simulink model "IBDC_DAB_SC"  (R2020b)
settings: Solver=VariableStepAuto  StartTime=0.0  StopTime=0.2  MaxStep=5.0E-7  RelTol=1e-3
values from neighbouring files (symbols this model uses):
  L = 19.5e-6    (= 1.95e-05)    [Initialize.m]
  P = 1/f    (= 4e-06)    [Initialize.m]
  R_load = 115.8    [Initialize.m]
  Sample = 1e-8    (= 1e-08)    [Initialize.m]
  Vref = 340    [Initialize.m]
libraries: powerlib x32, powerlib_meascontrol x6, pid_lib x2, electricdrivelib x1
settings Model: Creator=reigs  LastModifiedBy=reigs
settings SolverCC: DecoupledContinuousIntegration=on

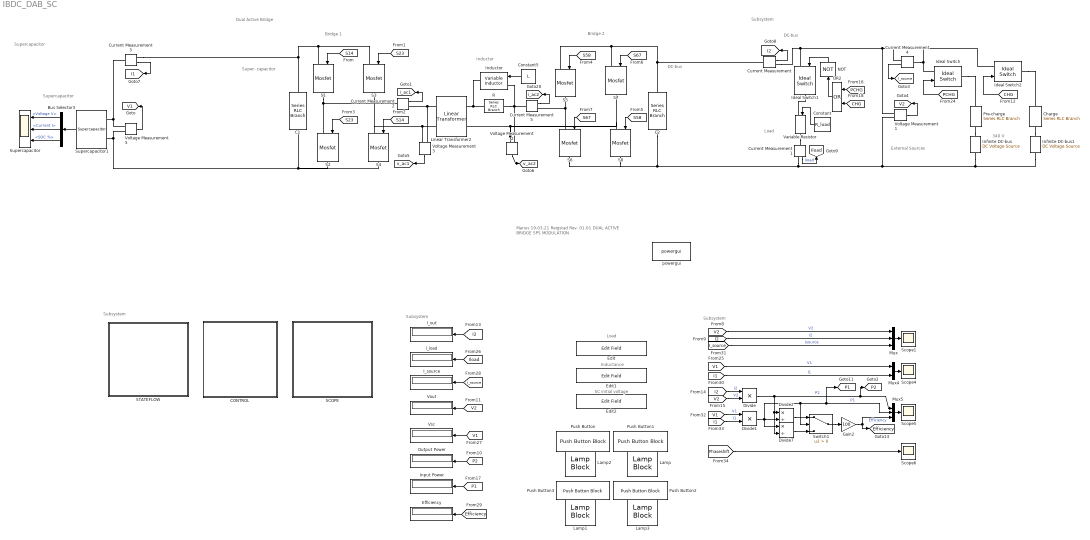
== system IBDC_DAB_SC ==
  note: Subsystem
  note: Dual Active Bridge
  note: Subsystem
  note: Subsystem
  note: Subsystem
  note: Supercapacitor
  note: Marius 19.03.21
      | Reigstad Rev. 01.01
      |
      | DUAL ACTIVE BRIDGE
      | SPS MODULATION
  note: Supercapacitor
  note: SC initial voltage
  note: Inductance
  note: Load
  note: Inductor
  note: Bridge 1
  note: Bridge 2
  note: DC-bus
  note: Super-
      | capacitor
  note: 340 V
  note: DC-bus
  note: External Sources
  note: Load
  " Inductor" : powerlib/Elements/Variable Inductor  methode=Backward Euler  Labsmin=1e-6  Initialize=off  iL0=0  L0=1e-3  Vl0=0
      settings: SourceProductBaseCode=PS
  Bus Selector3 : BusSelector  OutputSignals=Voltage V,Current I,SOC %
  C1 : powerlib/Elements/Series RLC Branch  LConnTagsString=__new0  RConnTagsString=__new0  BranchType=RC  Resistance=0.0032  Inductance=1e-3  SetiL0=off  InitialCurrent=0  Capacitance=500e-6  Setx0=on  InitialVoltage=Vsc  Measurements=None
  C2 : powerlib/Elements/Series RLC Branch  LConnTagsString=__new0  RConnTagsString=__new0  BranchType=RC  Resistance=0.0000001  Inductance=1e-3  SetiL0=off  InitialCurrent=0  Capacitance=54e-6  Setx0=off  InitialVoltage=340  Measurements=None
  CONTROL : Subsystem
  Charge : powerlib/Elements/Series RLC Branch  LConnTagsString=__new0  RConnTagsString=__new0  BranchType=R  Resistance=2  Inductance=1e-3  SetiL0=off  InitialCurrent=0  Capacitance=500e-6  Setx0=off  InitialVoltage=340  Measurements=None
  Constant : Constant  Value=R_load
  Constant5 : Constant  Value=L
  Current Measurement{,1..5} (6 alike) : powerlib/Measurements/Current Measurement  PhasorSimulation=off  OutputType=Complex  PSBequivalent=0
  Divide : Product  Inputs=**
  Divide1 : Product  Inputs=**
  Divide2 : Product  Inputs=*/
  Divide7 : Product  Inputs=*/
  Edit : EditField  LabelPosition=Hide  ShowInitialText=on  Alignment=Center
  Edit1 : EditField  LabelPosition=Hide  ShowInitialText=on  Alignment=Center
  Edit2 : EditField  LabelPosition=Hide  ShowInitialText=on  Alignment=Center
  Efficiency : Display
  Gain2 : Gain  Gain=100
  I_load : Display
  I_out : Display
  I_source : Display
  Ideal Switch : powerlib/Power Electronics/Ideal Switch  Ron=0.001  Lon=0  IC=0  Rs=1e5  Cs=inf  Measurements=off
  Ideal Switch1 : powerlib/Power Electronics/Ideal Switch  Ron=0.001  Lon=0  IC=0  Rs=1e5  Cs=inf  Measurements=off
  Ideal Switch2 : powerlib/Power Electronics/Ideal Switch  Ron=0.001  Lon=0  IC=0  Rs=1e5  Cs=inf  Measurements=off
  Infinite DC-bus : powerlib/Electrical Sources/DC Voltage Source  Amplitude=Vref  Measurements=None
  Infinite DC-bus1 : powerlib/Electrical Sources/DC Voltage Source  Amplitude=Vref  Measurements=None
  Input Power : Display
  Lamp{,1..3} (4 alike) : LampBlock
  Linear Transformer2 : powerlib/Elements/Linear Transformer  UNITS=SI  NominalPower=[2000 250000]  winding1=[180 0.0324 8.2505e-07]  winding2=[340 0.1156 2.9438e-06]  ThreeWindings=off  winding3=[3.15e+05 99225 2.5267]  RmLm=[8100 0.0051565]  Measurements=None  DataType=on
  Mux : Mux  Inputs=3
  Mux4 : Mux  Inputs=2
  Mux5 : Mux  Inputs=3
  NOT : Logic  Operator=NOT  IconShape=distinctive  AllPortsSameDT=off  OutDataTypeStr=boolean
  OR2 : Logic  Operator=OR  IconShape=distinctive  AllPortsSameDT=off  OutDataTypeStr=boolean
  Output Power : Display
  Pre-charge : powerlib/Elements/Series RLC Branch  LConnTagsString=__new0  RConnTagsString=__new0  BranchType=R  Resistance=30  Inductance=1e-3  SetiL0=off  InitialCurrent=0  Capacitance=500e-6  Setx0=off  InitialVoltage=340  Measurements=None
  Push Button : PushButtonBlock  ButtonText=STOP
  Push Button1 : PushButtonBlock  ButtonText=CHARGE
  Push Button2 : PushButtonBlock  ButtonText=STABILIZE
  Push Button3 : PushButtonBlock  ButtonText=PRECHARGE
  R : powerlib/Elements/Series RLC Branch  LConnTagsString=__new0  RConnTagsString=__new0  BranchType=R  Resistance=1e9  Inductance=1e-3  SetiL0=off  InitialCurrent=0  Capacitance=54.3e-6  Setx0=on  InitialVoltage=167  Measurements=None
  S{1..8} (8 alike) : powerlib/Power Electronics/Mosfet  Ron=ron_mosfet_pri  Lon=0  Rd=ron_body_diode_pri  Vfd=vf_body_diode_pri  IC=0  Rs=1e5  Cs=inf  Measurements=off
  SCOPE : Subsystem
  STATEFLOW : Subsystem
  Scope{1,4..6} (4 alike) : Scope
  Supercapacitor : Scope  NumInputPorts=3
  Supercapacitor1 : electricdrivelib/Extra Sources/Supercapacitor  C=5  Rdc=230.4e-3  Voltage=180  Ns=72  Np=1  Vinit=Vsc  Temp=25  PresetModel=off  EstParam=off  Nc=1  r=1e-9  epsilon=6.0208e-10  Ich=10  Vstern="[0.161  2.7  7.8]"  Self_dis=on  Ioc=10  Vself="[48  47.8  47.06  44.65]"  demandeplot=off  I="[5.55  6.25  ]"  Units=sec  Vmax=0  If=0  deltaV=0  alpha=0  sec=0
      settings: SourceProductBaseCode=PS
  Switch1 : Switch  Criteria=u2 > Threshold
  Variable Resistor : powerlib/Elements/Variable Resistor  Rabsmin=1e-3
      settings: SourceProductBaseCode=PS
  Voltage Measurement{1..3,5} (4 alike) : powerlib/Measurements/Voltage Measurement  PhasorSimulation=off  OutputType=Complex  PSBequivalent=0
  Vout : Display
  Vsc : Display
  powergui : powerlib/powergui  Priority=1  SimulationMode=Discrete  SampleTime=1e-8  frequency=60  Iterations=50  frequencyindice=0  Pbase=100e6  ErrMax=1e-4  UnitsV=kV  UnitsW=MW  buscounter=0  FunctionMessages=off  echomessages=off  EnableUseOfTLC=off  CurrentSourceSwitches=off  DisableSnubberDevices=off  DisableRonSwitches=off  DisableVfSwitches=off  DisplayEquations=off  AutomaticDiscreteSolvers=off  SolverType=Tustin/Backward Euler (TBE)  Interpol=off  ExternalGateDelay=off  methode=off  Ts=100  x0status=blocks  SPID=on  SwTol=0  HookPort=off  NonlinearTolerance=1e-4  nMaxIteration=100  ContinueOnMaxIteration=off  RestoreLinks=warning  ResistiveCurrentMeasurement=off  Frange=[0:2:500]  Ylog=off  Xlog=on  ShowGrid=off  save=off  variable=ZData  structure=0  ZoomFFT=off  StartTime=0.0  cycles=1  DisplayStyle=1  fundamental=60  FreqAxis=off  MaxFrequency=1000  frequencyindicesteady=1  RmsSteady=1  display=off
  tag scope: Efficiency=global, I1=global, I2=global, I_source=global, Iload=global, P1=global, P2=global, V1=global, V2=global, i_ac1=global, i_ac2=global, v_ac1=global, v_ac2=global
  wires:
  Current Measurement3/1 -> [I1]
  Supercapacitor1/1 -> Bus Selector3/1
  Voltage Measurement5/1 -> [V1]
  Bus Selector3/3 -> Supercapacitor/3  "<SOC %>"
  Bus Selector3/1 -> Supercapacitor/1  "<Voltage V>"
  Bus Selector3/2 -> Supercapacitor/2  "<Current I>"
  [P2] -> Output Power/1
  [Efficiency] -> Efficiency/1
  [I_source] -> I_source/1
  [V2] -> Vout/1
  [P1] -> Input Power/1
  [I2] -> I_out/1
  [Iload] -> I_load/1
  [V1] -> Vsc/1
  [I2] -> Divide/1  "I2"
  [I1] -> Divide1/2  "I1"
  Mux4/1 -> Scope4/1
  [I_source] -> Mux/3  "Isource"
  [I2] -> Mux/2  "I2"
  [Phaseshift] -> Scope6/1
  [V2] -> Mux/1  "V2"
  [I1] -> Mux4/2  "I1"
  Divide1/1 -> Switch1/2, Mux5/2, [P1], Divide2/2, Divide7/1  "P1"
  Mux/1 -> Scope1/1
  [V2] -> Divide/2  "V2"
  [V1] -> Mux4/1  "V1"
  Gain2/1 -> Mux5/3, [Efficiency]  "Efficiency"
  [V1] -> Divide1/1  "V1"
  Mux5/1 -> Scope5/1
  Divide/1 -> Divide7/2, Divide2/1, Mux5/1, [P2]  "P2"
  Switch1/1 -> Gain2/1
  Divide7/1 -> Switch1/3
  Divide2/1 -> Switch1/1
  [S58] -> S5/1
  [S14] -> S4/1
  [S67] -> S6/1
  Voltage Measurement2/1 -> [v_ac2]
  Voltage Measurement3/1 -> [v_ac1]
  [S23] -> S3/1
  [S67] -> S7/1
  [S58] -> S8/1
  Current Measurement2/1 -> [i_ac1]
  Current Measurement5/1 -> [i_ac2]
  [S23] -> S2/1
  [S14] -> S1/1
  Constant5/1 -> " Inductor"/1
  NOT/1 -> Ideal Switch1/1
  Current Measurement4/1 -> [I_source]
  [PCHG] -> OR2/1
  OR2/1 -> NOT/1
  [PCHG] -> Ideal Switch/1
  [CHG] -> OR2/2
  [CHG] -> Ideal Switch2/1
  Constant/1 -> Variable Resistor/1
  Voltage Measurement1/1 -> [V2]
  Current Measurement/1 -> [I2]
  Current Measurement1/1 -> [Iload]  "Iload"
  connections:
  Current Measurement3/LConn1 -- Voltage Measurement5/LConn1 -- Supercapacitor1/LConn1
  S1/RConn1 -- S2/LConn1 -- Current Measurement2/LConn1
  S1/LConn1 -- Current Measurement3/RConn1 -- C1/LConn1 -- S3/LConn1
  Voltage Measurement3/LConn2 -- Linear Transformer2/LConn2 -- S3/RConn1 -- S4/LConn1
  Supercapacitor1/LConn2 -- S4/RConn1 -- S2/RConn1 -- C1/RConn1 -- Voltage Measurement5/LConn2
  Current Measurement5/LConn1 -- R/LConn1 -- Voltage Measurement2/LConn1 -- " Inductor"/LConn1
  R/RConn1 -- " Inductor"/RConn1 -- Linear Transformer2/RConn1
  S6/LConn1 -- S5/RConn1 -- Current Measurement5/RConn1
  Voltage Measurement2/LConn2 -- S8/LConn1 -- S7/RConn1 -- Linear Transformer2/RConn2
  Voltage Measurement3/LConn1 -- Linear Transformer2/LConn1 -- Current Measurement2/RConn1
  Infinite DC-bus/LConn1 -- Infinite DC-bus1/LConn1 -- S6/RConn1 -- S8/RConn1 -- C2/RConn1 -- Current Measurement1/RConn1 -- Voltage Measurement1/LConn2
  Charge/RConn1 -- Infinite DC-bus1/RConn1
  C2/LConn1 -- Current Measurement/LConn1 -- S7/LConn1 -- S5/LConn1
  Ideal Switch1/RConn1 -- Variable Resistor/LConn1
  Current Measurement4/LConn1 -- Ideal Switch/LConn1 -- Ideal Switch2/LConn1
  Variable Resistor/RConn1 -- Current Measurement1/LConn1
  Pre-charge/RConn1 -- Infinite DC-bus/RConn1
  Ideal Switch/RConn1 -- Pre-charge/LConn1
  Ideal Switch2/RConn1 -- Charge/LConn1
  Current Measurement/RConn1 -- Ideal Switch1/LConn1 -- Voltage Measurement1/LConn1 -- Current Measurement4/RConn1

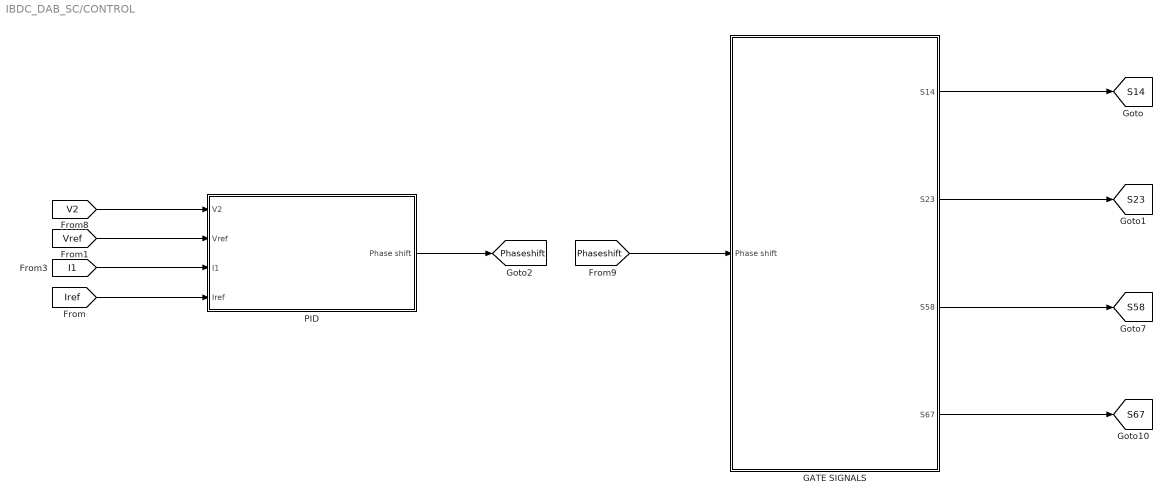
== system IBDC_DAB_SC/CONTROL ==
  GATE SIGNALS : Subsystem
  PID : Subsystem
  tag scope: Phaseshift=global, S14=global, S23=global, S58=global, S67=global
  wires:
  [Phaseshift] -> GATE SIGNALS/1(Phase shift)
  [V2] -> PID/1(V2)
  [Vref] -> PID/2(Vref)
  GATE SIGNALS/1(S14) -> [S14]
  GATE SIGNALS/2(S23) -> [S23]
  GATE SIGNALS/3(S58) -> [S58]
  GATE SIGNALS/4(S67) -> [S67]
  PID/1(Phase shift) -> [Phaseshift]
  [I1] -> PID/3(I1)
  [Iref] -> PID/4(Iref)

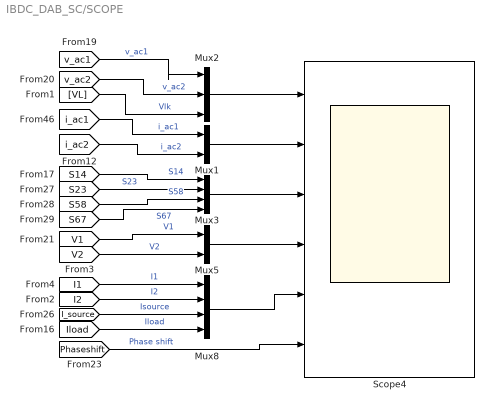
== system IBDC_DAB_SC/SCOPE ==
  Mux1 : Mux  Inputs=2
  Mux2 : Mux  Inputs=3
  Mux3 : Mux
  Mux5 : Mux  Inputs=2
  Mux8 : Mux
  Scope4 : Scope  NumInputPorts=6
  wires:
  [VL] -> Mux2/3  "Vlk"
  Mux2/1 -> Scope4/1
  [v_ac1] -> Mux2/1  "v_ac1"
  [I1] -> Mux8/1  "I1"
  [v_ac2] -> Mux2/2  "v_ac2"
  [I_source] -> Mux8/3  "Isource"
  [S67] -> Mux3/4  "S67"
  [i_ac2] -> Mux1/2  "i_ac2"
  [S14] -> Mux3/1  "S14"
  [Iload] -> Mux8/4  "Iload"
  [S58] -> Mux3/3  "S58"
  [i_ac1] -> Mux1/1  "i_ac1"
  Mux8/1 -> Scope4/5
  [S23] -> Mux3/2  "S23"
  Mux1/1 -> Scope4/2
  Mux3/1 -> Scope4/3
  [Phaseshift] -> Scope4/6  "Phase shift"
  [I2] -> Mux8/2  "I2"
  [V2] -> Mux5/2  "V2"
  Mux5/1 -> Scope4/4
  [V1] -> Mux5/1  "V1"

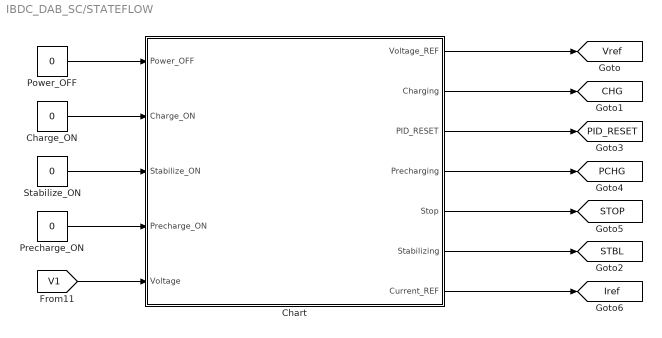
== system IBDC_DAB_SC/STATEFLOW ==
  Charge_ON : Constant  Value=0
  Chart : Stateflow chart  TreatAsAtomicUnit=on
  Power_OFF : Constant  Value=0
  Precharge_ON : Constant  Value=0
  Stabilize_ON : Constant  Value=0
  tag scope: CHG=global, Iref=global, PCHG=global, PID_RESET=global, STBL=global, STOP=global, Vref=global
  wires:
  Power_OFF/1 -> Chart/1(Power_OFF)
  [V1] -> Chart/5(Voltage)
  Charge_ON/1 -> Chart/2(Charge_ON)
  Stabilize_ON/1 -> Chart/3(Stabilize_ON)
  Precharge_ON/1 -> Chart/4(Precharge_ON)
  Chart/1(Voltage_REF) -> [Vref]
  Chart/5(Stop) -> [STOP]
  Chart/4(Precharging) -> [PCHG]
  Chart/3(PID_RESET) -> [PID_RESET]
  Chart/2(Charging) -> [CHG]
  Chart/6(Stabilizing) -> [STBL]
  Chart/7(Current_REF) -> [Iref]

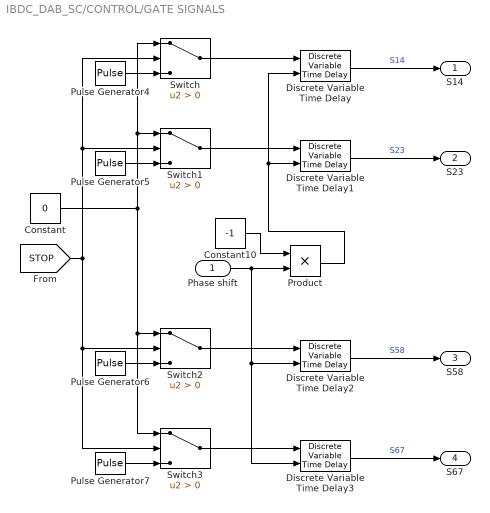
== system IBDC_DAB_SC/CONTROL/GATE SIGNALS ==
  Phase shift : Inport
  Constant : Constant  Value=0
  Constant10 : Constant  Value=-1
  Discrete Variable Time Delay{,1..3} (4 alike) : powerlib_meascontrol/Additional Components/Discrete Variable Time Delay  MaxDelay=1  InitialValue=0  Ts=Sample  DFT=on
      settings: SourceProductBaseCode=PS
  Product : Product
  Pulse Generator4 : DiscretePulseGenerator  PulseType=Time based  Period=P  PulseWidth=49  VectorParams1D=off
  Pulse Generator5 : DiscretePulseGenerator  PulseType=Time based  Period=P  PulseWidth=49  PhaseDelay=P/2  VectorParams1D=off
  Pulse Generator6 : DiscretePulseGenerator  PulseType=Time based  Period=P  PulseWidth=49
  Pulse Generator7 : DiscretePulseGenerator  PulseType=Time based  Period=P  PulseWidth=49  PhaseDelay=P/2
  Switch{,1..3} (4 alike) : Switch  Criteria=u2 > Threshold
  S14 : Outport
  S23 : Outport  Port=2
  S58 : Outport  Port=3
  S67 : Outport  Port=4
  wires:
  Phase shift/1 -> Product/2, Discrete Variable Time Delay2/2, Discrete Variable Time Delay3/2
  Discrete Variable Time Delay3/1 -> S67/1  "S67"
  Switch3/1 -> Discrete Variable Time Delay3/1
  Switch1/1 -> Discrete Variable Time Delay1/1
  Constant10/1 -> Product/1
  Switch2/1 -> Discrete Variable Time Delay2/1
  Discrete Variable Time Delay2/1 -> S58/1  "S58"
  Discrete Variable Time Delay/1 -> S14/1  "S14"
  Discrete Variable Time Delay1/1 -> S23/1  "S23"
  Switch/1 -> Discrete Variable Time Delay/1
  Product/1 -> Discrete Variable Time Delay/2, Discrete Variable Time Delay1/2
  Pulse Generator7/1 -> Switch3/3
  [STOP] -> Switch/2, Switch1/2, Switch3/2, Switch2/2
  Pulse Generator6/1 -> Switch2/3
  Pulse Generator5/1 -> Switch1/3
  Pulse Generator4/1 -> Switch/3
  Constant/1 -> Switch3/1, Switch2/1, Switch/1, Switch1/1

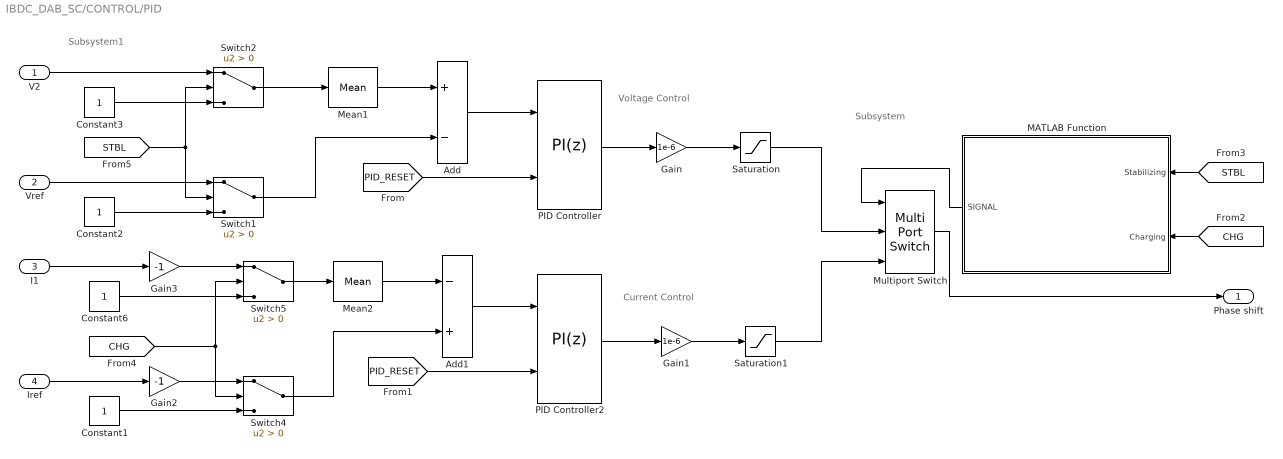
== system IBDC_DAB_SC/CONTROL/PID ==
  note: Subsystem1
  note: Subsystem
  note: Voltage Control
  note: Current Control
  V2 : Inport
  Vref : Inport  Port=2
  I1 : Inport  Port=3
  Iref : Inport  Port=4
  Add : Sum  Inputs=+-
  Add1 : Sum  Inputs=-+
  Constant{1..3,6} (4 alike) : Constant
  Gain : Gain  Gain=1e-6
  Gain1 : Gain  Gain=1e-6
  Gain2 : Gain  Gain=-1
  Gain3 : Gain  Gain=-1
  MATLAB Function : MATLAB Function  TreatAsAtomicUnit=on
  Mean1 : powerlib_meascontrol/Measurements/Mean  Freq=250000  Vinit=0  Ts=Sample
  Mean2 : powerlib_meascontrol/Measurements/Mean  Freq=250000  Vinit=0  Ts=Sample
  Multiport Switch : MultiPortSwitch  Inputs=2
  PID Controller : pid_lib/PID Controller  Controller=PI  Form=Parallel  TimeDomain=Discrete-time  UseExternalTs=off  SampleTime=Sample  IntegratorMethod=Forward Euler  FilterMethod=Forward Euler  ControllerParametersSource=internal  P=-0.0035  I=-2.4900  D=0  UseFilter=on  N=100  TunerSelectOption=Transfer Function Based (PID Tuner App)  InitialConditionSource=internal  InitialConditionForIntegrator=0  InitialConditionForFilter=0  DifferentiatorICPrevScaledInput=0  ExternalReset=rising  TrackingMode=off  Kt=1  LimitOutput=off  SatLimitsSource=internal  UpperSaturationLimit=2e-6  LowerSaturationLimit=-2e-6  LinearizeAsGain=on  AntiWindupMode=none  Kb=1  POutMin=[]  POutMax=[]  IOutMin=[]  IOutMax=[]  DOutMin=[]  DOutMax=[]  NOutMin=[]  NOutMax=[]  SumOutMin=[]  SumOutMax=[]  SaturationOutMin=[]  SaturationOutMax=[]  PParamMin=[]  PParamMax=[]  IParamMin=[]  IParamMax=[]  DParamMin=[]  DParamMax=[]  NParamMin=[]  NParamMax=[]  KbParamMin=[]  KbParamMax=[]  KtParamMin=[]  KtParamMax=[]  KbOutMin=[]  KbOutMax=[]  KtOutMin=[]  KtOutMax=[]  IntegratorOutMin=[]  IntegratorOutMax=[]  FilterOutMin=[]  FilterOutMax=[]  SumI1OutMin=[]  SumI1OutMax=[]  SumI2OutMin=[]  SumI2OutMax=[]  SumI3OutMin=[]  SumI3OutMax=[]  SumI4OutMin=[]  SumI4OutMax=[]  SumDOutMin=[]  SumDOutMax=[]  DifferentiatorOutMin=[]  DifferentiatorOutMax=[]  FilterDiffOutCoefMin=[]  FilterDiffOutCoefMax=[]  ReciprocalOutMin=[]  ReciprocalOutMax=[]  SumDenOutMin=[]  SumDenOutMax=[]  SumNumOutMin=[]  SumNumOutMax=[]  DivideOutMin=[]  DivideOutMax=[]  UdiffTsProdOutMin=[]  UdiffTsProdOutMax=[]  NTsProdOutMin=[]  NTsProdOutMax=[]  UintegralTsProdOutMin=[]  UintegralTsProdOutMax=[]  UngainTsProdOutMin=[]  UngainTsProdOutMax=[]  IntegratorContinuousStateAttributes=''  IntegratorStateMustResolveToSignalObject=off  IntegratorRTWStateStorageClass=Auto  FilterContinuousStateAttributes=''  FilterStateMustResolveToSignalObject=off  FilterRTWStateStorageClass=Auto  ParallelPVariant=InternalParameters  IdealPVariant=Disabled  IVariant=InternalParameters  DVariant=Disabled  IntegratorVariant=Discrete  SatVariant=Disabled  AWVariant=Passthrough  PCopyVariant=Disabled  TRVariant=Disabled  FdbkBlocksVariant=Forward  IdealPFdbkVariant=Disabled  SatFdbkVariant=Disabled  DerivativeFilterVariant=Disabled  NVariant=Disabled  NCopyVariant=Disabled_SignalSpec  FilterICVariant=Disabled  IntegratorICVariant=InternalICs  ExternalResetVariant=ExternalReset  TRSumVariant=Passthrough  SumFdbkVariant=Disabled  SumVariant=Sum_PI  TsampFilterVariant=InternalTs  TsampNgainVariant=Passthrough  TsampIntegralVariant=Passthrough  ExternalSaturationOutDataTypeStr=Inherit: Same as second input
  PID Controller2 : pid_lib/PID Controller  Controller=PI  Form=Parallel  TimeDomain=Discrete-time  UseExternalTs=off  SampleTime=Sample  IntegratorMethod=Forward Euler  FilterMethod=Forward Euler  ControllerParametersSource=internal  P=-0.01  I=-100  D=0  UseFilter=on  N=100  TunerSelectOption=Transfer Function Based (PID Tuner App)  InitialConditionSource=internal  InitialConditionForIntegrator=0  InitialConditionForFilter=0  DifferentiatorICPrevScaledInput=0  ExternalReset=rising  TrackingMode=off  Kt=1  LimitOutput=off  SatLimitsSource=internal  UpperSaturationLimit=2e-6  LowerSaturationLimit=-2e-6  LinearizeAsGain=on  AntiWindupMode=none  Kb=1  POutMin=[]  POutMax=[]  IOutMin=[]  IOutMax=[]  DOutMin=[]  DOutMax=[]  NOutMin=[]  NOutMax=[]  SumOutMin=[]  SumOutMax=[]  SaturationOutMin=[]  SaturationOutMax=[]  PParamMin=[]  PParamMax=[]  IParamMin=[]  IParamMax=[]  DParamMin=[]  DParamMax=[]  NParamMin=[]  NParamMax=[]  KbParamMin=[]  KbParamMax=[]  KtParamMin=[]  KtParamMax=[]  KbOutMin=[]  KbOutMax=[]  KtOutMin=[]  KtOutMax=[]  IntegratorOutMin=[]  IntegratorOutMax=[]  FilterOutMin=[]  FilterOutMax=[]  SumI1OutMin=[]  SumI1OutMax=[]  SumI2OutMin=[]  SumI2OutMax=[]  SumI3OutMin=[]  SumI3OutMax=[]  SumI4OutMin=[]  SumI4OutMax=[]  SumDOutMin=[]  SumDOutMax=[]  DifferentiatorOutMin=[]  DifferentiatorOutMax=[]  FilterDiffOutCoefMin=[]  FilterDiffOutCoefMax=[]  ReciprocalOutMin=[]  ReciprocalOutMax=[]  SumDenOutMin=[]  SumDenOutMax=[]  SumNumOutMin=[]  SumNumOutMax=[]  DivideOutMin=[]  DivideOutMax=[]  UdiffTsProdOutMin=[]  UdiffTsProdOutMax=[]  NTsProdOutMin=[]  NTsProdOutMax=[]  UintegralTsProdOutMin=[]  UintegralTsProdOutMax=[]  UngainTsProdOutMin=[]  UngainTsProdOutMax=[]  IntegratorContinuousStateAttributes=''  IntegratorStateMustResolveToSignalObject=off  IntegratorRTWStateStorageClass=Auto  FilterContinuousStateAttributes=''  FilterStateMustResolveToSignalObject=off  FilterRTWStateStorageClass=Auto  ParallelPVariant=InternalParameters  IdealPVariant=Disabled  IVariant=InternalParameters  DVariant=Disabled  IntegratorVariant=Discrete  SatVariant=Disabled  AWVariant=Passthrough  PCopyVariant=Disabled  TRVariant=Disabled  FdbkBlocksVariant=Forward  IdealPFdbkVariant=Disabled  SatFdbkVariant=Disabled  DerivativeFilterVariant=Disabled  NVariant=Disabled  NCopyVariant=Disabled_SignalSpec  FilterICVariant=Disabled  IntegratorICVariant=InternalICs  ExternalResetVariant=ExternalReset  TRSumVariant=Passthrough  SumFdbkVariant=Disabled  SumVariant=Sum_PI  TsampFilterVariant=InternalTs  TsampNgainVariant=Passthrough  TsampIntegralVariant=Passthrough  ExternalSaturationOutDataTypeStr=Inherit: Same as second input
  Saturation : Saturate  UpperLimit=2e-6  LowerLimit=-2e-6
  Saturation1 : Saturate  UpperLimit=2e-6  LowerLimit=-2e-6
  Switch{1..2,4..5} (4 alike) : Switch  Criteria=u2 > Threshold
  Phase shift : Outport
  wires:
  Multiport Switch/1 -> Phase shift/1
  Saturation1/1 -> Multiport Switch/3
  Saturation/1 -> Multiport Switch/2
  [STBL] -> MATLAB Function/1(Stabilizing)
  MATLAB Function/1(SIGNAL) -> Multiport Switch/1
  [CHG] -> MATLAB Function/2(Charging)
  V2/1 -> Switch2/1
  I1/1 -> Gain3/1
  [CHG] -> Switch4/2, Switch5/2
  Add/1 -> PID Controller/1
  PID Controller2/1 -> Gain1/1
  Gain1/1 -> Saturation1/1
  [PID_RESET] -> PID Controller2/2
  Constant1/1 -> Switch4/3
  Vref/1 -> Switch1/1
  Gain/1 -> Saturation/1
  [PID_RESET] -> PID Controller/2
  Mean1/1 -> Add/1
  Add1/1 -> PID Controller2/1
  Constant3/1 -> Switch2/3
  Gain3/1 -> Switch5/1
  [STBL] -> Switch1/2, Switch2/2
  Switch5/1 -> Mean2/1
  PID Controller/1 -> Gain/1
  Constant2/1 -> Switch1/3
  Iref/1 -> Gain2/1
  Gain2/1 -> Switch4/1
  Switch4/1 -> Add1/2
  Switch2/1 -> Mean1/1
  Mean2/1 -> Add1/1
  Constant6/1 -> Switch5/3
  Switch1/1 -> Add/2

== matlab function IBDC_DAB_SC/CONTROL/PID/MATLAB Function ==
  data: Stabilizing input; Charging input; SIGNAL output
function SIGNAL  = pidSELECTOR(Stabilizing,Charging)


if (Charging==1)
    SIGNAL = 2;

else 
    SIGNAL = 1;
end

== stateflow chart IBDC_DAB_SC/STATEFLOW/Chart ==
  state Charge
    en: Charging = true;
    en: PID_RESET = true;
    en: Current_REF = -6.25;
    ex: Charging = false;
    ex: PID_RESET = false;
  state Power_OFF
    en: Voltage_REF = 0;
    en: Current_REF = 0;
    en: Stop = true;
  state Precharge
    en: Precharging = true;
    ex: Precharging = false;
    ex: Stop = false;
  state Stabilize
    en: Stabilizing = true;
    en: PID_RESET = true;
    en: Voltage_REF = 340;
    ex: Stabilizing = false;
    ex: PID_RESET = false;
  Charge -> Power_OFF [order 1] : [Power_OFF]
  Precharge -> Charge [order 1] : [Charge_ON && ...
      |  ~Stabilize_ON]
  Charge -> Stabilize [order 2] : [Stabilize_ON && ...
      | ~Charge_ON]
  Stabilize -> Charge [order 2] : [Charge_ON && ...
      | ~Stabilize_ON]
  Power_OFF -> Precharge : [Precharge_ON && ...
      | ~Power_OFF]
  (default) -> Power_OFF
  Precharge -> Power_OFF [order 2] : [Power_OFF]
  Precharge -> Stabilize [order 3] : [Stabilize_ON && ...
      |    ~Charge_ON]
  Stabilize -> Power_OFF [order 1] : [Power_OFF || Voltage < 90]
  data: Power_OFF input; Charge_ON input; Stabilize_ON input; Precharge_ON input; Voltage input; Voltage_REF output; Charging output; PID_RESET output; Precharging output; Stop output; Stabilizing output; Current_REF output
